simulink library "aab"  (Simulink 8.1)
settings: Solver=ode45  StartTime=0.0  StopTime=10.0  RelTol=1e-3
settings Model: Creator=xsellart  LastModifiedBy=AT015086

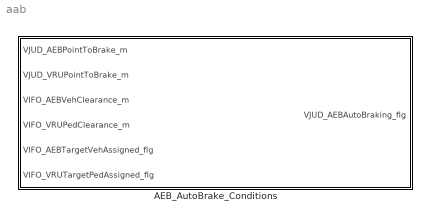
== system aab ==
  AEB_AutoBrake_Conditions : Subsystem

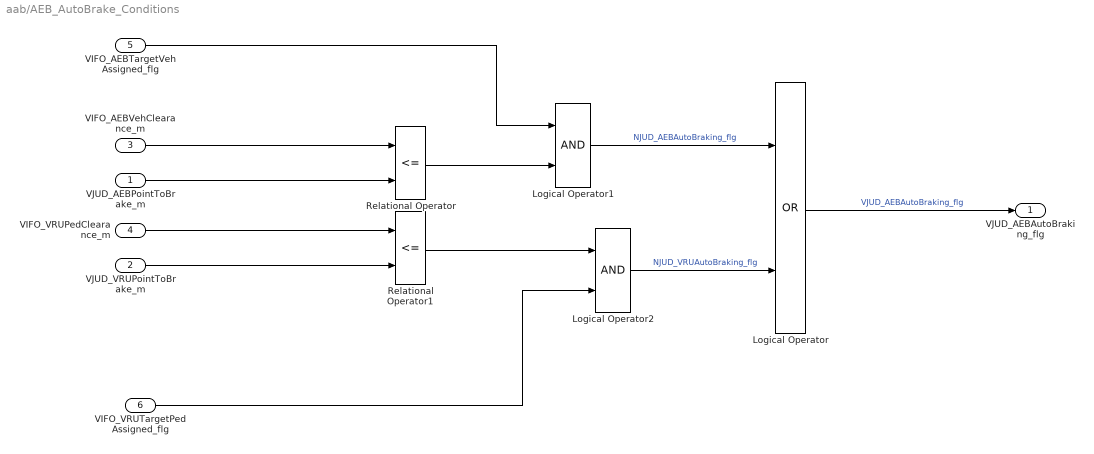
== system aab/AEB_AutoBrake_Conditions ==
  VJUD_AEBPointToBrake_m : Inport
  VJUD_VRUPointToBrake_m : Inport  Port=2
  VIFO_AEBVehClearance_m : Inport  Port=3
  VIFO_VRUPedClearance_m : Inport  Port=4
  VIFO_AEBTargetVehAssigned_flg : Inport  Port=5
  VIFO_VRUTargetPedAssigned_flg : Inport  Port=6
  Logical Operator : Logic  Operator=OR  AllPortsSameDT=off  OutDataTypeStr=boolean
  Logical Operator1 : Logic  AllPortsSameDT=off  OutDataTypeStr=boolean
  Logical Operator2 : Logic  AllPortsSameDT=off  OutDataTypeStr=boolean
  Relational Operator : RelationalOperator  Operator=<=  OutDataTypeStr=boolean
  Relational Operator1 : RelationalOperator  Operator=<=  OutDataTypeStr=boolean
  VJUD_AEBAutoBraking_flg : Outport
  wires:
  Logical Operator/1 -> VJUD_AEBAutoBraking_flg/1  "VJUD_AEBAutoBraking_flg"
  VIFO_AEBVehClearance_m/1 -> Relational Operator/1
  VJUD_AEBPointToBrake_m/1 -> Relational Operator/2
  VIFO_VRUPedClearance_m/1 -> Relational Operator1/1
  VJUD_VRUPointToBrake_m/1 -> Relational Operator1/2
  Relational Operator/1 -> Logical Operator1/2
  Relational Operator1/1 -> Logical Operator2/1
  Logical Operator1/1 -> Logical Operator/1  "NJUD_AEBAutoBraking_flg"
  VIFO_AEBTargetVehAssigned_flg/1 -> Logical Operator1/1
  Logical Operator2/1 -> Logical Operator/2  "NJUD_VRUAutoBraking_flg"
  VIFO_VRUTargetPedAssigned_flg/1 -> Logical Operator2/2
